simulink library "TYPEBP_MASTER_tmp"  (Simulink 8.6)
settings: Solver=ode45  StartTime=0.0  StopTime=10.0  RelTol=1e-3
undefined symbols (not defined in the file): TYPEC, TYPEC_MASTER
libraries: cdsEpicsOut x112, cdsFilt x79, cdsTP x59, cdsFiltCtrl x36, VIS_LIB x20, cdsEpicsIn x18, cdsMuxMatrix x14, STATE_BIO_MASTER x12, cdsEpicsBinIn x8, cdsFunctionCall x4, lockin x4, cdsEpicsStringIn x2
(part 7 of 13)

== system TYPEBP_MASTER_tmp/TYPEBPMASTER_TEST/BF/TEST ==
  GAS : cdsFilt/Subsystem  Tag=cdsFilt  Description=|
      | Purpose:                                                                                                                                                                                                                                  
      | Standard CDS IIR filter module.                                                                                                                                                                                                           
      |                                                                                                                                                                                                                                           
      | Operation:                                                                                                                                                                                                                                
      | Consists of 10 second order section IIR filters, plus a ramped gain stage. In FE code, also provides pre-defined test points and excitation channel inputs. The filter coefficients are defined in the LIGO system using the 'foton' tool.
      |                                                                                                                                                                                                                                           
      | Usage:                                                                                                                                                                                                                                    
      | Name the part with the desired filter module name.
      settings: AttributesFormatString=%<Tag>
  Ground{1..8} (8 alike) : Ground
  L : cdsFilt/Subsystem  Tag=cdsFilt  Description=|
      | Purpose:                                                                                                                                                                                                                                  
      | Standard CDS IIR filter module.                                                                                                                                                                                                           
      |                                                                                                                                                                                                                                           
      | Operation:                                                                                                                                                                                                                                
      | Consists of 10 second order section IIR filters, plus a ramped gain stage. In FE code, also provides pre-defined test points and excitation channel inputs. The filter coefficients are defined in the LIGO system using the 'foton' tool.
      |                                                                                                                                                                                                                                           
      | Usage:                                                                                                                                                                                                                                    
      | Name the part with the desired filter module name.
      settings: AttributesFormatString=%<Tag>
  P : cdsFilt/Subsystem  Tag=cdsFilt  Description=|
      | Purpose:                                                                                                                                                                                                                                  
      | Standard CDS IIR filter module.                                                                                                                                                                                                           
      |                                                                                                                                                                                                                                           
      | Operation:                                                                                                                                                                                                                                
      | Consists of 10 second order section IIR filters, plus a ramped gain stage. In FE code, also provides pre-defined test points and excitation channel inputs. The filter coefficients are defined in the LIGO system using the 'foton' tool.
      |                                                                                                                                                                                                                                           
      | Usage:                                                                                                                                                                                                                                    
      | Name the part with the desired filter module name.
      settings: AttributesFormatString=%<Tag>
  R : cdsFilt/Subsystem  Tag=cdsFilt  Description=|
      | Purpose:                                                                                                                                                                                                                                  
      | Standard CDS IIR filter module.                                                                                                                                                                                                           
      |                                                                                                                                                                                                                                           
      | Operation:                                                                                                                                                                                                                                
      | Consists of 10 second order section IIR filters, plus a ramped gain stage. In FE code, also provides pre-defined test points and excitation channel inputs. The filter coefficients are defined in the LIGO system using the 'foton' tool.
      |                                                                                                                                                                                                                                           
      | Usage:                                                                                                                                                                                                                                    
      | Name the part with the desired filter module name.
      settings: AttributesFormatString=%<Tag>
  STATUS : cdsEpicsBinIn/Subsystem  Tag=cdsEpicsBinIn  Description=|
      | Purpose:                                                                            
      | Create an EPICS binary (0 or 1) input channel to the FE realtime controls.          
      |                                                                                     
      | Operation:                                                                          
      | Outputs value from an EPICS ai record. Value is binary input (bi Epics record type).
      |                                                                                     
      | Usage:                                                                              
      | Name the part with the desired EPICS channel name.
      settings: AttributesFormatString=%<Tag>
  T : cdsFilt/Subsystem  Tag=cdsFilt  Description=|
      | Purpose:                                                                                                                                                                                                                                  
      | Standard CDS IIR filter module.                                                                                                                                                                                                           
      |                                                                                                                                                                                                                                           
      | Operation:                                                                                                                                                                                                                                
      | Consists of 10 second order section IIR filters, plus a ramped gain stage. In FE code, also provides pre-defined test points and excitation channel inputs. The filter coefficients are defined in the LIGO system using the 'foton' tool.
      |                                                                                                                                                                                                                                           
      | Usage:                                                                                                                                                                                                                                    
      | Name the part with the desired filter module name.
      settings: AttributesFormatString=%<Tag>
  V : cdsFilt/Subsystem  Tag=cdsFilt  Description=|
      | Purpose:                                                                                                                                                                                                                                  
      | Standard CDS IIR filter module.                                                                                                                                                                                                           
      |                                                                                                                                                                                                                                           
      | Operation:                                                                                                                                                                                                                                
      | Consists of 10 second order section IIR filters, plus a ramped gain stage. In FE code, also provides pre-defined test points and excitation channel inputs. The filter coefficients are defined in the LIGO system using the 'foton' tool.
      |                                                                                                                                                                                                                                           
      | Usage:                                                                                                                                                                                                                                    
      | Name the part with the desired filter module name.
      settings: AttributesFormatString=%<Tag>
  Y : cdsFilt/Subsystem  Tag=cdsFilt  Description=|
      | Purpose:                                                                                                                                                                                                                                  
      | Standard CDS IIR filter module.                                                                                                                                                                                                           
      |                                                                                                                                                                                                                                           
      | Operation:                                                                                                                                                                                                                                
      | Consists of 10 second order section IIR filters, plus a ramped gain stage. In FE code, also provides pre-defined test points and excitation channel inputs. The filter coefficients are defined in the LIGO system using the 'foton' tool.
      |                                                                                                                                                                                                                                           
      | Usage:                                                                                                                                                                                                                                    
      | Name the part with the desired filter module name.
      settings: AttributesFormatString=%<Tag>
  LONG_Out : Outport
  TRANS_Out : Outport  Port=2
  VERT_Out : Outport  Port=3
  ROLL_Out : Outport  Port=4
  PITCH_Out : Outport  Port=5
  YAW_Out : Outport  Port=6
  GAS_Out : Outport  Port=7
  wires:
  Ground8/1 -> GAS/1
  GAS/1 -> GAS_Out/1
  Ground7/1 -> STATUS/1
  Ground4/1 -> R/1
  Ground5/1 -> P/1
  Ground6/1 -> Y/1
  Ground3/1 -> V/1
  Ground2/1 -> T/1
  Ground1/1 -> L/1
  R/1 -> ROLL_Out/1
  P/1 -> PITCH_Out/1
  Y/1 -> YAW_Out/1
  V/1 -> VERT_Out/1
  T/1 -> TRANS_Out/1
  L/1 -> LONG_Out/1

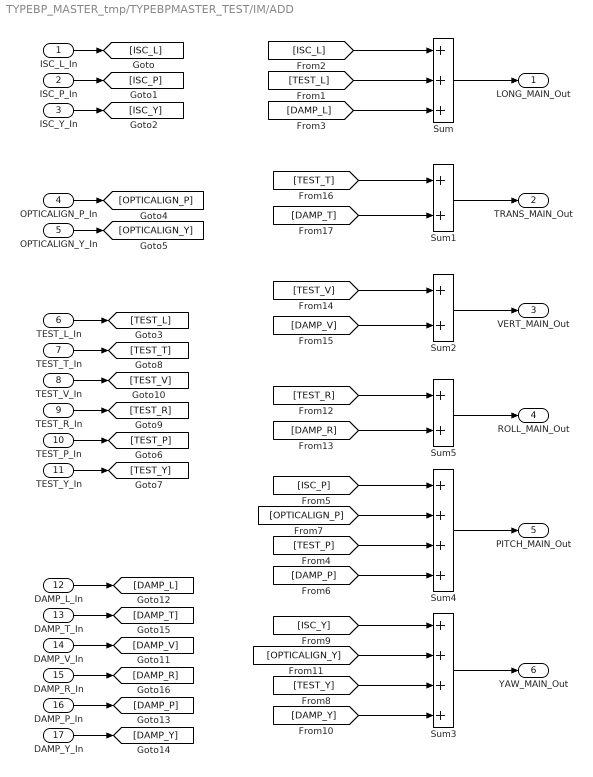
== system TYPEBP_MASTER_tmp/TYPEBPMASTER_TEST/IM/ADD ==
  ISC_L_In : Inport
  ISC_P_In : Inport  Port=2
  ISC_Y_In : Inport  Port=3
  OPTICALIGN_P_In : Inport  Port=4
  OPTICALIGN_Y_In : Inport  Port=5
  TEST_L_In : Inport  Port=6
  TEST_T_In : Inport  Port=7
  TEST_V_In : Inport  Port=8
  TEST_R_In : Inport  Port=9
  TEST_P_In : Inport  Port=10
  TEST_Y_In : Inport  Port=11
  DAMP_L_In : Inport  Port=12
  DAMP_T_In : Inport  Port=13
  DAMP_V_In : Inport  Port=14
  DAMP_R_In : Inport  Port=15
  DAMP_P_In : Inport  Port=16
  DAMP_Y_In : Inport  Port=17
  Sum : Sum  Inputs=+++
  Sum1 : Sum
  Sum2 : Sum
  Sum3 : Sum  Inputs=++++
  Sum4 : Sum  Inputs=++++
  Sum5 : Sum
  LONG_MAIN_Out : Outport
  TRANS_MAIN_Out : Outport  Port=2
  VERT_MAIN_Out : Outport  Port=3
  ROLL_MAIN_Out : Outport  Port=4
  PITCH_MAIN_Out : Outport  Port=5
  YAW_MAIN_Out : Outport  Port=6
  wires:
  [DAMP_V] -> Sum2/2
  [TEST_V] -> Sum2/1
  [DAMP_T] -> Sum1/2
  [TEST_T] -> Sum1/1
  [DAMP_R] -> Sum5/2
  [TEST_R] -> Sum5/1
  [DAMP_Y] -> Sum3/4
  [TEST_Y] -> Sum3/3
  [OPTICALIGN_Y] -> Sum3/2
  [ISC_Y] -> Sum3/1
  [DAMP_P] -> Sum4/4
  [TEST_P] -> Sum4/3
  [OPTICALIGN_P] -> Sum4/2
  [ISC_P] -> Sum4/1
  DAMP_Y_In/1 -> [DAMP_Y]
  DAMP_P_In/1 -> [DAMP_P]
  DAMP_R_In/1 -> [DAMP_R]
  DAMP_V_In/1 -> [DAMP_V]
  DAMP_T_In/1 -> [DAMP_T]
  DAMP_L_In/1 -> [DAMP_L]
  TEST_Y_In/1 -> [TEST_Y]
  TEST_P_In/1 -> [TEST_P]
  TEST_R_In/1 -> [TEST_R]
  TEST_V_In/1 -> [TEST_V]
  TEST_T_In/1 -> [TEST_T]
  TEST_L_In/1 -> [TEST_L]
  ISC_Y_In/1 -> [ISC_Y]
  ISC_P_In/1 -> [ISC_P]
  ISC_L_In/1 -> [ISC_L]
  OPTICALIGN_Y_In/1 -> [OPTICALIGN_Y]
  OPTICALIGN_P_In/1 -> [OPTICALIGN_P]
  Sum1/1 -> TRANS_MAIN_Out/1
  Sum2/1 -> VERT_MAIN_Out/1
  Sum5/1 -> ROLL_MAIN_Out/1
  [DAMP_L] -> Sum/3
  [TEST_L] -> Sum/2
  [ISC_L] -> Sum/1
  Sum/1 -> LONG_MAIN_Out/1
  Sum3/1 -> YAW_MAIN_Out/1
  Sum4/1 -> PITCH_MAIN_Out/1

== system TYPEBP_MASTER_tmp/TYPEBPMASTER_TEST/IM/ADD_LKIN ==
  LKN_V1_In : Inport
  LKN_V2_In : Inport  Port=2
  LKIN_V3_In : Inport  Port=3
  LKIN_H1_In : Inport  Port=4
  LKIN_H2_In : Inport  Port=5
  LKIN_H3_In : Inport  Port=6
  OSEM_V1_In : Inport  Port=7
  OSEM_V2_In : Inport  Port=8
  OSEM_V3_In : Inport  Port=9
  OSEM_H1_In : Inport  Port=10
  OSEM_H2_In : Inport  Port=11
  OSEM_H3_In : Inport  Port=12
  Sum{,1..5} (6 alike) : Sum
  V1_Out : Outport
  V2_Out : Outport  Port=2
  V3_Out : Outport  Port=3
  H1_Out : Outport  Port=4
  H2_Out : Outport  Port=5
  H3_Out : Outport  Port=6
  wires:
  LKIN_H3_In/1 -> Sum2/1
  LKIN_H2_In/1 -> Sum5/1
  Sum5/1 -> H2_Out/1
  OSEM_H2_In/1 -> Sum5/2
  Sum2/1 -> H3_Out/1
  OSEM_H3_In/1 -> Sum2/2
  LKIN_H1_In/1 -> Sum1/1
  LKIN_V3_In/1 -> Sum3/1
  LKN_V2_In/1 -> Sum4/1
  Sum/1 -> V1_Out/1
  LKN_V1_In/1 -> Sum/1
  OSEM_V1_In/1 -> Sum/2
  Sum3/1 -> V3_Out/1
  Sum4/1 -> V2_Out/1
  OSEM_V3_In/1 -> Sum3/2
  OSEM_V2_In/1 -> Sum4/2
  Sum1/1 -> H1_Out/1
  OSEM_H1_In/1 -> Sum1/2
